simulink model "H8_1GDL_currentinput_ecuaciones"  (R2022b)
settings: Solver=VariableStepAuto  StartTime=0.0  StopTime=10  RelTol=1e-3
model workspace (MAT data in the model file):
  surfaceBlockParameters = Simulink.LookupTable
  surfaceBlockParameters.Table = Simulink.lookuptable.Table
  surfaceBlockParameters.Table.Value = [145.669360614  122.326612109  101.996418654  84.6787802495  70.3736968941  59.0811685884  50.8011953324  45.5337771261  43.2789139695  44.0366058625; 185.313749978  156.270189263  130.473313595  107.923122972  88.6196173961  72.5627968658  59.7526613816  50.1892109434  43.8724455513  40.8023652052; 237.482290208  203.298417321  172.595359476  145.373116673  121.631688913  101.371076195  84.59127852  71.2922958872  61.4741282968  55.1367757489; 296.780859506  258.017174483  222.968434498  191.634639553  164.015789646  140.111884779  119.92292495  103.44891016  90.6898404082  81.6457156957; 357.815336073  315.032338952  276.198416866  241.313569815  210.377797799  183.391100818  160.353478873  141.264931963  126.125460088  114.935063248; 415.191598113  368.94978893  326.891184779  289.01578566  255.323591572  225.814602516  200.488818491  179.346239498  162.386865537  149.610696607; 463.515523826  414.37540262  369.652616441  329.347165291  293.459049169  261.988268074  234.934822007  212.298710969  194.079934958  180.278493975; 497.392991416  445.915058223  399.088590054  356.91358691  319.39004879  286.517975694  258.297367623  234.728224576  215.810546553  201.544333555; 511.429879083  458.174633941  409.804983819  366.320928719  327.722468638  294.009603579  265.18233354  241.240658522  222.184578525  208.014093548]
  surfaceBlockParameters.Table.Dimensions = [9 10]
  surfaceBlockParameters.Table.DataType = 'auto'
  surfaceBlockParameters.Table.FieldName = 'Table_force'
  surfaceBlockParameters.Breakpoints(1) = Simulink.lookuptable.Breakpoint
  surfaceBlockParameters.Breakpoints(1).Value = [-40 -31.1 -22.2 -13.3 -4.4 4.5 13.4 22.3 31.2]
  surfaceBlockParameters.Breakpoints(1).TunableSizeName = 'N1'
  surfaceBlockParameters.Breakpoints(1).Dimensions = [1 9]
  surfaceBlockParameters.Breakpoints(1).DataType = 'auto'
  surfaceBlockParameters.Breakpoints(1).FieldName = 'BP1_current'
  surfaceBlockParameters.Breakpoints(2) = Simulink.lookuptable.Breakpoint
  surfaceBlockParameters.Breakpoints(2).Value = [0.011 0.0123 0.0136 0.0149 0.0162 0.0175 0.0188 0.0201 0.0214 0.0227]
  surfaceBlockParameters.Breakpoints(2).TunableSizeName = 'N2'
  surfaceBlockParameters.Breakpoints(2).Dimensions = [1 10]
  surfaceBlockParameters.Breakpoints(2).DataType = 'auto'
  surfaceBlockParameters.Breakpoints(2).FieldName = 'BP2_airgap'
  surfaceBlockParameters.AllowMultipleInstancesOfTypeToHaveDifferentTableBreakpointSizes = 0
  surfaceBlockParameters.SupportTunableSize = 0
  surfaceBlockParameters.StructTypeInfo = Simulink.lookuptable.StructTypeInfo
  surfaceBlockParameters.StructTypeInfo.Name = 'surfaceBlockParameters_type'
  surfaceBlockParameters.StructTypeInfo.DataScope = 'Auto'
values from neighbouring files (symbols this model uses):
  g = 9.81    [hemsH8.m]
  m = i    [barrido_masas.m]    (also in hemsH8.m = 200)
settings Model: Creator=USUARIO  LastModifiedBy=ramuj

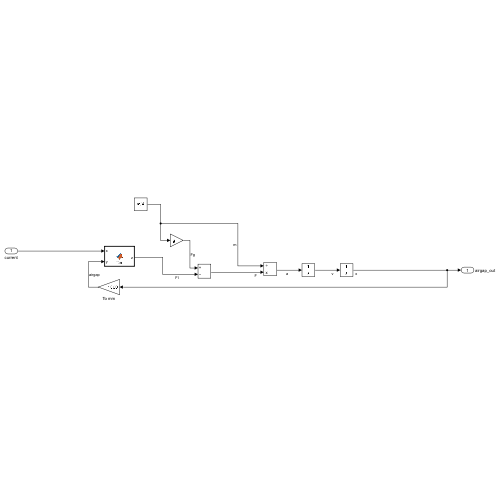
[thumbnail: Simulink's stored preview of the top-level diagram]
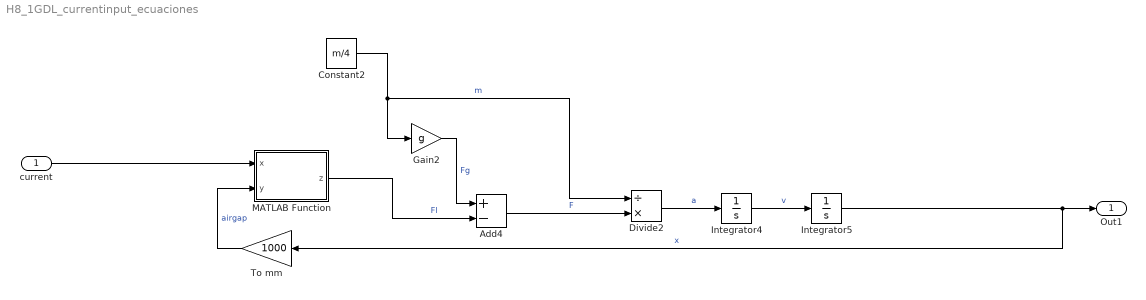
== system H8_1GDL_currentinput_ecuaciones ==
  current : Inport
  Add4 : Sum  Inputs=+-
  Constant2 : Constant  Value=m/4
  Divide2 : Product  Inputs=/*
  Gain2 : Gain  Gain=g
  Integrator4 : Integrator
  Integrator5 : Integrator  InitialCondition=0.01905
  MATLAB Function : MATLAB Function  TreatAsAtomicUnit=on
  To mm : Gain  Gain=1000
  Out1 : Outport  SignalName=airgap_out
  wires:
  Gain2/1 -> Add4/1  "Fg"
  Integrator5/1 -> Out1/1, To mm/1  "x"
  MATLAB Function/1(z) -> Add4/2  "Fl"
  Add4/1 -> Divide2/2  "F"
  Divide2/1 -> Integrator4/1  "a"
  Constant2/1 -> Gain2/1, Divide2/1  "m"
  Integrator4/1 -> Integrator5/1  "v"
  To mm/1 -> MATLAB Function/2(y)  "airgap"
  current/1 -> MATLAB Function/1(x)

== matlab function H8_1GDL_currentinput_ecuaciones/MATLAB Function ==
  data: x input; z output; y input
function z = fcn(x, y)

p00 =        1730;
p10 =       18.31;
p01 =      -88.01;
p20 =     0.02748;
p11 =     -0.4182;
p02 =       1.476;

z = p00 + p10*x + p01*y + p20*x^2 + p11*x*y + p02*y^2;
